simulink library "droop_controller_lib"
settings: Solver=ode45  StartTime=0.0  StopTime=10.0  RelTol=1e-3
values from neighbouring files (symbols this model uses):
  Droop_control_time_step = Ts    (= 8e-05)    [global_parameters.m]
  f = 60    [global_parameters.m]
undefined symbols (not defined in the file or in its folder): filter_a, filter_b, filter_c, filter_d, pd_filt_init
settings Model: Creator=CH24070  LastModifiedBy=CH24070

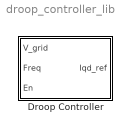
== system droop_controller_lib ==
  Droop Controller : Subsystem  mask(D and Q axis droop controller){Kdroop_Q=0, Kdroop_P=-10e3/5, VacRMS=480, IacRMS=100, filter_co=2e6}
      mask prompts: Kdroop_Q "Reactive Power Droop Gain"; Kdroop_P "Real Power Droop Gain"; VacRMS "Nominal AC Voltage RMS"; IacRMS "Maximum Current RMS"; filter_co "Filter Cut Off Frequency (Hz)"
      mask help: Droop Controller for controlling D and Q axis current based on grid frequency and voltage.
      mask init:
      | global_parameters
      | droop_control_init
      mask Help:
      | Real Power Droop Gain- Ratio of Watts to Hz for injecting power to the grid in response to frequency changes.
      | Reactive Power Droop Gain- Ratio of kVars to RMS volts for injecting reactive power to the grid.
      | Grid Tie Line to Neutral Voltage- RMS voltage for the grid tie interface.
      | Maximum Current RMS- Maximum current that can be injected to the grid.
      | Droop Filter Cut Off- Fastest frequency that will be responded to for injecting power to the grid.

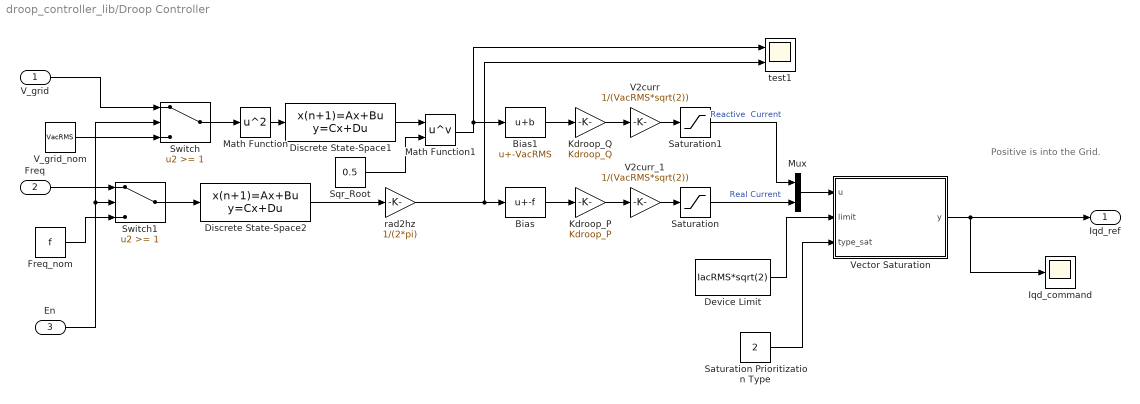
== system droop_controller_lib/Droop Controller ==
  note: Positive is into the Grid.
  V_grid : Inport
  Freq : Inport  Port=2
  En : Inport  Port=3
  Bias : Bias  Bias=-f
  Bias1 : Bias  Bias=-VacRMS
  Device Limit : Constant  Value=IacRMS*sqrt(2)
  Discrete State-Space1 : DiscreteStateSpace  A=filter_a  B=filter_b  C=filter_c  D=filter_d  X0=pd_filt_init  SampleTime=Droop_control_time_step
  Discrete State-Space2 : DiscreteStateSpace  A=filter_a  B=filter_b  C=filter_c  D=filter_d  SampleTime=Droop_control_time_step
  Freq_nom : Constant  Value=f
  Iqd_command : Scope
      settings: YMin=-750  YMax=750
  Kdroop_P : Gain  Gain=Kdroop_P
  Kdroop_Q : Gain  Gain=Kdroop_Q
  Math Function : Math  Operator=square  OutputSignalType=real  SaturateOnIntegerOverflow=on
  Math Function1 : Math  Operator=pow  SaturateOnIntegerOverflow=on
  Mux : Mux  Inputs=2
  Saturation : Saturate  UpperLimit=IacRMS*sqrt(2)  LowerLimit=-IacRMS*sqrt(2)
  Saturation Prioritization Type : Constant  Value=2
  Saturation1 : Saturate  UpperLimit=IacRMS*sqrt(2)  LowerLimit=-IacRMS*sqrt(2)
  Sqr_Root : Constant  Value=0.5
  Switch : Switch  Threshold=1
  Switch1 : Switch  Threshold=1
  V2curr : Gain  Gain=1/(VacRMS*sqrt(2))
  V2curr_1 : Gain  Gain=1/(VacRMS*sqrt(2))
  V_grid_nom : Constant  Value=VacRMS
  Vector Saturation : MATLAB Function  TreatAsAtomicUnit=on
  rad2hz : Gain  Gain=1/(2*pi)
  test1 : Scope  NumInputPorts=2
      settings: YMin=479.5~58.95  YMax=486~59.06
  Iqd_ref : Outport
  wires:
  V2curr/1 -> Saturation1/1
  Saturation Prioritization Type/1 -> Vector Saturation/3(type_sat)
  rad2hz/1 -> test1/2, Bias/1
  Kdroop_P/1 -> V2curr_1/1
  V2curr_1/1 -> Saturation/1
  Device Limit/1 -> Vector Saturation/2(limit)
  Mux/1 -> Vector Saturation/1(u)
  Bias/1 -> Kdroop_P/1
  Kdroop_Q/1 -> V2curr/1
  Vector Saturation/1(y) -> Iqd_ref/1, Iqd_command/1
  Discrete State-Space2/1 -> rad2hz/1
  Saturation1/1 -> Mux/1  "Reactive  Current"
  Saturation/1 -> Mux/2  "Real Current"
  Math Function1/1 -> test1/1, Bias1/1
  Bias1/1 -> Kdroop_Q/1
  Math Function/1 -> Discrete State-Space1/1
  Sqr_Root/1 -> Math Function1/2
  Discrete State-Space1/1 -> Math Function1/1
  Switch/1 -> Math Function/1
  V_grid/1 -> Switch/1
  V_grid_nom/1 -> Switch/3
  Switch1/1 -> Discrete State-Space2/1
  Freq_nom/1 -> Switch1/3
  Freq/1 -> Switch1/1
  En/1 -> Switch/2, Switch1/2

== matlab function droop_controller_lib/Droop Controller/Vector Saturation ==
  data: u input; y output; limit input; type_sat input
function y = fcn(u, limit, type_sat)
% When the magnitude is of u is greater than limit prioritize the
% saturation to u(type_sat) dimension.  u is two dimensional input.
%#codegen
y=zeros(2,1); % required initialization
u_sign=sign(u);

if(abs(u(1)) > limit)
    u(1) = u_sign(1).*limit;
end
if(abs(u(2)) > limit)
    u(2) =  u_sign(2).*limit;
end
if(u(1)^2 + u(2)^2 > limit^2)
    if(type_sat == 1) % priority given to u(1)
        y(1) = u(1);
        y(2) = u_sign(2) .* sqrt(limit^2 - u(1)^2); 
    else  % priority given to u(2)
        y(2) = u(2);
        y(1) =  u_sign(1) .* sqrt(limit^2 - u(2)^2); 
    end
else
    y = u;
end
